simulink model "TestRapidAcc"  (R2024a)
settings: Solver=VariableStepAuto  StartTime=0.0  StopTime=10.0  RelTol=1e-3
settings Model: Creator=eunice.duplessis  LastModifiedBy=eunice.duplessis

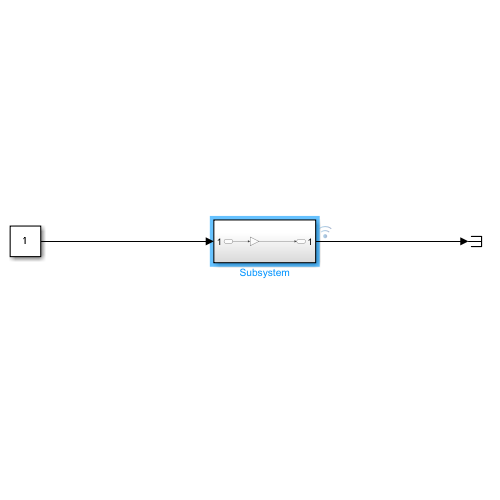
[thumbnail: Simulink's stored preview of the top-level diagram]
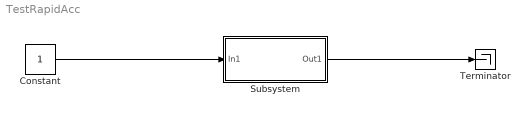
== system TestRapidAcc ==
  Constant : Constant
  Subsystem : Subsystem
  Terminator : Terminator
  wires:
  Constant/1 -> Subsystem/1(In1)
  Subsystem/1(Out1) -> Terminator/1

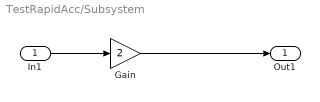
== system TestRapidAcc/Subsystem ==
  In1 : Inport
  Gain : Gain  Gain=2
  Out1 : Outport
  wires:
  In1/1 -> Gain/1
  Gain/1 -> Out1/1
